simulink model "sim1"  (Simulink 6.3)
settings: Solver=ode45  StartTime=0.0  StopTime=70  RelTol=1e-3
settings Model: LastModifiedBy=Usuario  StrictBusMsg=None

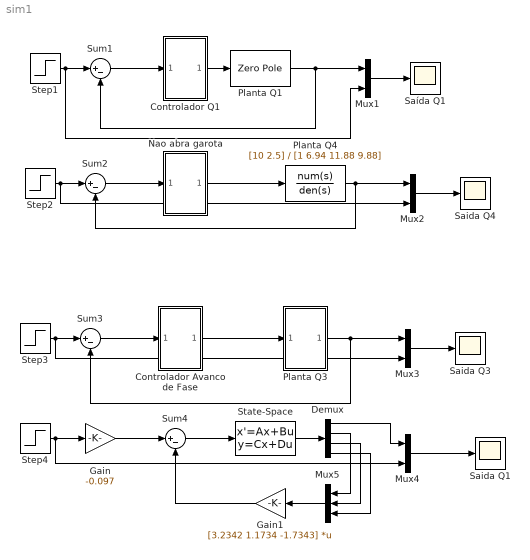
== system sim1 ==
  Controlador Avanco de Fase : Subsystem  mask{K=0.0593, a=4.7192, T=1.7964}
      mask prompts: K "Ganho K"; a "Parâmetro a < 1"; T "Parâmetro T"
  Controlador Q1 : Subsystem  mask{K1=0.99, K2=0.42, K3=0.9071}
      mask prompts: K1 "Ganho K1 (proporcional)"; K2 "Ganho K2 (derivativo)"; K3 "Ganho K3 (integral)"
  Demux : Demux
  Gain : Gain  Gain=-0.097
  Gain1 : Gain  Orientation=left  Gain=[3.2342 1.1734 -1.7343]  Multiplication=Matrix(K*u) (u vector)
  Mux{1..4} (4 alike) : Mux  Inputs=2
  Mux5 : Mux  Orientation=left  Inputs=3
  Nao abra garota : Subsystem  mask{K=0.9172, K2=1.6644}
      mask prompts: K "Ganho Proporcional (K)"; K2 "Ganho Integral (K2)"
  Planta Q1 : ZeroPole  Zeros=[]  Poles=[0 -1 -3.94]  Gain=[49.4]
  Planta Q3 : Subsystem
  Planta Q4 : TransferFcn  Numerator=[10 2.5]  Denominator=[1 6.94 11.88 9.88]
  Saida Q1 : Scope
      settings: SaveName=ScopeData3
  Saida Q3 : Scope
  Saida Q4 : Scope
      settings: SaveName=ScopeData2
  Saída Q1 : Scope
      settings: YMin=5.55112e-017  YMax=1
  State-Space : StateSpace  A=[0 1 0; 3.94 1 1; -2 0 1]  B=[0;8.5;1]  C=[1 0 8.5; 1 0 0; 0 1 0; 0 0 1]  D=[0;0;0;0]
  Step{1..4} (4 alike) : Step  SampleTime=0
  Sum{1..4} (4 alike) : Sum  Inputs=|+-
  wires:
  Step1/1 -> Sum1/1, Mux1/2
  Mux1/1 -> Saída Q1/1
  Planta Q1/1 -> Mux1/1, Sum1/2
  Controlador Q1/1(Out1) -> Planta Q1/1
  Sum1/1 -> Controlador Q1/1(In1)
  Step2/1 -> Sum2/1, Mux2/2
  Mux2/1 -> Saida Q4/1
  Planta Q4/1 -> Mux2/1, Sum2/2
  Nao abra garota/1(Out1) -> Planta Q4/1
  Sum2/1 -> Nao abra garota/1(In1)
  Step3/1 -> Sum3/1, Mux3/2
  Mux3/1 -> Saida Q3/1
  Planta Q3/1(Out1) -> Mux3/1, Sum3/2
  Controlador Avanco de Fase/1(Out1) -> Planta Q3/1(In1)
  Sum3/1 -> Controlador Avanco de Fase/1(In1)
  Step4/1 -> Mux4/2, Gain/1
  Mux4/1 -> Saida Q1/1
  Gain/1 -> Sum4/1
  Sum4/1 -> State-Space/1
  Gain1/1 -> Sum4/2
  State-Space/1 -> Demux/1
  Demux/1 -> Mux4/1
  Mux5/1 -> Gain1/1
  Demux/2 -> Mux5/1
  Demux/3 -> Mux5/2
  Demux/4 -> Mux5/3

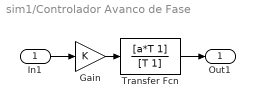
== system sim1/Controlador Avanco de Fase ==
  In1 : Inport
  Gain : Gain  Gain=K
  Transfer Fcn : TransferFcn  Numerator=[a*T 1]  Denominator=[T 1]
  Out1 : Outport
  wires:
  Gain/1 -> Transfer Fcn/1
  In1/1 -> Gain/1
  Transfer Fcn/1 -> Out1/1

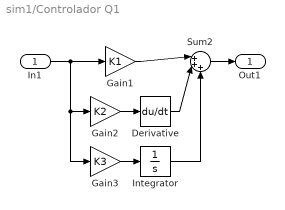
== system sim1/Controlador Q1 ==
  In1 : Inport
  Derivative : Derivative
  Gain1 : Gain  Gain=K1
  Gain2 : Gain  Gain=K2
  Gain3 : Gain  Gain=K3
  Integrator : Integrator
  Sum2 : Sum  Inputs=|+++
  Out1 : Outport
  wires:
  In1/1 -> Gain2/1, Gain3/1, Gain1/1
  Gain2/1 -> Derivative/1
  Gain1/1 -> Sum2/1
  Derivative/1 -> Sum2/2
  Gain3/1 -> Integrator/1
  Integrator/1 -> Sum2/3
  Sum2/1 -> Out1/1

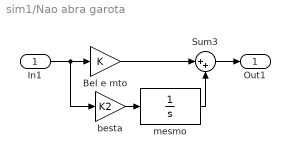
== system sim1/Nao abra garota ==
  In1 : Inport
  Bel e mto : Gain  Gain=K
  Sum3 : Sum  Inputs=|++
  besta : Gain  Gain=K2
  mesmo : TransferFcn  Denominator=[1 0]
  Out1 : Outport
  wires:
  In1/1 -> besta/1, Bel e mto/1
  besta/1 -> mesmo/1
  Bel e mto/1 -> Sum3/1
  mesmo/1 -> Sum3/2
  Sum3/1 -> Out1/1

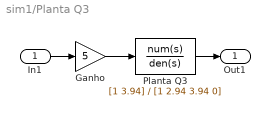
== system sim1/Planta Q3 ==
  In1 : Inport
  Ganho : Gain  Gain=5
  Planta Q3 : TransferFcn  Numerator=[1 3.94]  Denominator=[1 2.94 3.94 0]
  Out1 : Outport
  wires:
  Ganho/1 -> Planta Q3/1
  In1/1 -> Ganho/1
  Planta Q3/1 -> Out1/1
